simulink model "vehicle_model"  (R2021b)
settings: Solver=ode23tb  StartTime=0  StopTime=181.45  FixedStep=1e-5  RelTol=2e-1
InitFcn:
  | param_v1_script;
  | Ts=0.01;
  | scenario_generator;
  | Regen_on=0;
  | v_nom=10;
  | load('eq_udds.mat')
  | %load('eq_nedc.mat')
values from neighbouring files (symbols this model uses):
  b = 1.504    [dynamics_wheel.m]    (also in param_v1_script.m = Simulink.Parameter)
  BattChargeMax = 4.8    [param_v1_script.m]
  Battery = struct    [param_v1_script.m]
  BattSocInit = 0.75    [param_v1_script.m]
  BattTempInit = 25    [param_v1_script.m]
  BrkPrsMax = 5.0E+6    (= 5000000)    [param_v1_script.m]
  car = vehicle(scenario,'ClassID',1,'Position',[x_ego y_ego 0], 'Yaw' ,0,     'Length',3,'Width',2,'Height',1.6)    [scenario_generator.m]
  curvature = (DX.*D2Y - DY.*D2X) ./(DX.^2+DY.^2).^(3/2)    [ref_generator.m]
  direction = ones(length(gradbp),1)    [ref_generator.m]
  disk_abore = 0.05    [param_v1_script.m]
  Eb_init = 54.28*1000*3600    (= 195408000)    [param_v1_script.m]
  efficiency_table = [86.7 86.7 86.7 86.7 86.7 86.7 86.7 86.7 86.7 86.7 86.7 86.7 86.7 86.7     86.7 ... (first row only)    [param_v1_script.m]
  eta_i = 1    [param_v1_script.m]
  gradbp = distbp    [ref_generator.m]
  Jmotor = Simulink.Parameter    [param_v1_script.m]
  k = Simulink.Parameter    [param_v1_script.m]
  L = 30000    [scenario_generator.m]
  losses_table = [0 0 0 0 0 0 0 0 0 0 0 0 0 0 0 ... (first row only)    [param_v1_script.m]
  m = 3152    [param_v1_script.m]
  MaxChrgCurrLim = Simulink.Parameter    [param_v1_script.m]
  MaxDchrgCurrLim = Simulink.Parameter    [param_v1_script.m]
  MinCellVoltDchrgCurrentLim_BP = [2.5; 2.75; 3]    [param_v1_script.m]
  MinCellVoltDchrgCurrentLim_Table = [0 0.5 1]    [param_v1_script.m]
  MotSpd = [0 1600 3200 4477.56 4800 6400 8000 9600 11200 12800 14400 16000            ]    [param_v1_script.m]
  MotTrq = [450 450 450 450 419.771162404874 314.828371803655 251.862697442924            209.885581202437 179.901926744946 157.414185901828 139.923720801625            125.931348721462]    [param_v1_script.m]
  mu_kinetic = 0.2    [param_v1_script.m]
  Nd = 12    [param_v1_script.m]
  Ndiff = Simulink.Parameter    [param_v1_script.m]
  Np_Module = 31    [param_v1_script.m]
  Ns_Module = 24    [param_v1_script.m]
  num_pads = 2    [param_v1_script.m]
  NumModules = 4    [param_v1_script.m]
  psi_o = thetaRefs(1)*(pi/180)    [ref_generator.m]
  RegenBrkCutOff = [0 1]    [param_v1_script.m]
  RegenBrkSpd_bpt = [5 9]    [param_v1_script.m]
  Rm = 0.177    [param_v1_script.m]
  rw = 0.419    [param_v1_script.m]
  scenario = drivingScenario('SampleTime',0.1','StopTime',60)    [scenario_generator.m]
  SOCInit = 0.75    [param_v1_script.m]
  SOE_init = SOCInit    (= 0.75)    [param_v1_script.m]
  T_eff_bp = [0 32.142857142857146 64.285714285714292 96.428571428571431              128.57142857142858 160.71428571428572 192.85714285714286 225              257.14285714285717 289.28571428571428 321.42857142857144 353.57142857142856              385.71428571428572 417.85714285714283 450]    [param_v1_script.m]
  thetaRefs = smooth(gradbp,thetaRef)    [ref_generator.m]
  threshld = 50    [scenario_generator.m]
  VEH = struct    [dynamics_wheel.m]
  w_eff_bp = [0 1600 3200 4477.56 4800 6400 8000 9600 11200 12800 14400 16000              ]    [param_v1_script.m]
  xRef2s = smooth(gradbp,xRef2)    [ref_generator.m]
  yRef2s = smooth(gradbp,yRef2)    [ref_generator.m]
undefined symbols (not defined in the file or in its folder): DiscIntNeverNeededParam, InertFrm
libraries: simulink x11, autolibsharedcoupling x10, autolibshared x5, autolibutils x4, autolibshareddiff x3, sharedtransform x3, vehdynlibdriver x3, simulink_extras x3, sharedTrackingLibrary x2, vehdynlibtirecommon x2, vehdynlibtire x2, vehdynlibdrivercommon x2
(part 2 of 6)

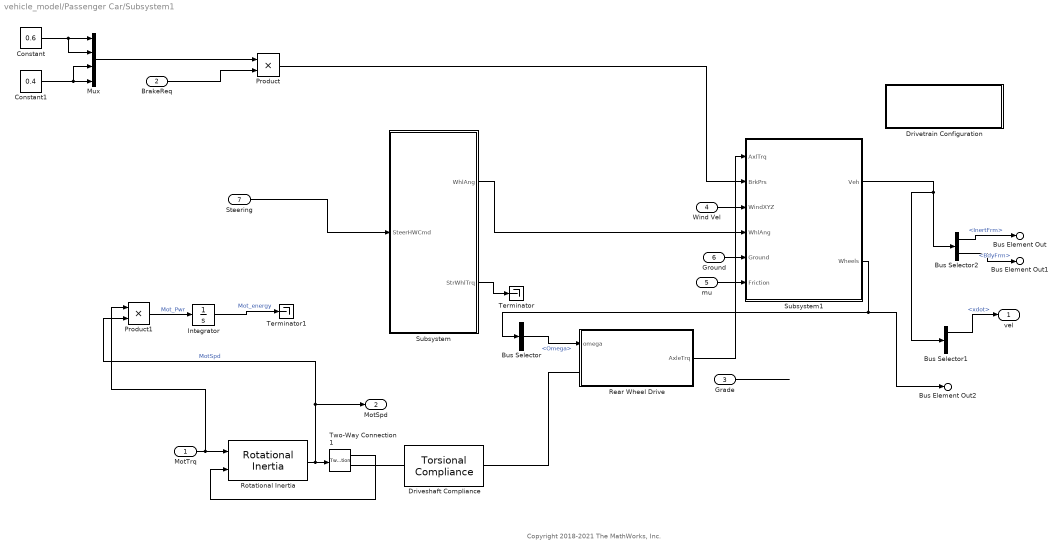
== system vehicle_model/Passenger Car/Subsystem1 ==
  note: Copyright 2018-2021 The MathWorks, Inc.
  MotTrq : Inport
  BrakeReq : Inport  Port=2
  Grade : Inport  Port=3
  Wind Vel : Inport  Port=4
  mu : Inport  Port=5
  Ground : Inport  Port=6
  Steering : Inport  Port=7
  Bus Selector : BusSelector  OutputSignals=TireFrame.Omega
  Bus Selector1 : BusSelector  OutputSignals=BdyFrm.Cg.Vel.xdot,BdyFrm.Cg.Vel.ydot
  Bus Selector2 : BusSelector  OutputSignals=InertFrm,BdyFrm
  Constant : Constant  Value=0.6
  Constant1 : Constant  Value=0.4
  Driveshaft Compliance : autolibsharedcoupling/Torsional Compliance  port_config=Two-way connection  extInfo=off  k=k  b=b  theta_o=theta_o  domega_o=domega_o  omega_c=omega_c  blkID=0  aMode=1
      settings: SourceProductBaseCode=PW,DR,MT,UV,VE
  Drivetrain Configuration : Subsystem  mask(Drivetrain Configuration){drivetrainMode=Rear Wheel Drive}
      mask prompts: drivetrainMode "Drivetrain Mode"
      mask help: Use this block to configure the dirvetrain mode.
      settings: AttributesFormatString=Active Mode: %<drivetrainMode>
      mask TypeOptions drivetrainMode: Front Wheel Drive | Rear Wheel Drive | All Wheel Drive
      mask Callback drivetrainMode:
      | switch get_param(gcb,'drivetrainMode')
      |     case 'Front Wheel Drive'
      |         set_param([bdroot '/Differential and Compliance'],'OverrideUsingVariant','0')
      |     case 'Rear Wheel Drive'
      |         set_param([bdroot '/Differential and Compliance'],'OverrideUsingVariant','1')
      |     case 'All Wheel Drive'
      |         set_param([bdroot '/Differential and Compliance'],'OverrideUsingVariant','2')
      |     otherwise
      |         set_param([bdroot '/Differential and Compliance'],'OverrideUsingVariant','0')
      | end
      mask Display: disp('Double click to configure drivetrain')
  Integrator : Integrator
  Mux : Mux
  Product : Product
  Product1 : Product
  Rear Wheel Drive : Subsystem  VariantControl=0
  Rotational Inertia : autolibsharedcoupling/Rotational Inertia  port_config=Simulink  extInfo=off  externJ=off  J=Jmotor  b=.001  omega_o=omega_o  blkID=0  aMode=1
      settings: SourceProductBaseCode=PW,DR,MT,UV,VE
  Subsystem : Subsystem
  Subsystem1 : Subsystem
  Terminator : Terminator
  Terminator1 : Terminator
  Two-Way Connection1 : TwoWayConnection
  vel : Outport  VectorParamsAs1DForOutWhenUnconnected=off
  MotSpd : Outport  Port=2  VectorParamsAs1DForOutWhenUnconnected=off  BusOutputAsStruct=on
  Bus Element Out : Outport  Port=3  PortName=Veh  Element=InertFrm
  Bus Element Out1 : Outport  Port=3  PortName=Veh  Element=BdyFrm
  Bus Element Out2 : Outport  Port=4  PortName=Wheels  Element=signal1
  wires:
  Subsystem/2(StrWhlTrq) -> Terminator/1
  Bus Selector/1 -> Rear Wheel Drive/1(omega)  "<Omega>"
  Rear Wheel Drive/1(AxleTrq) -> Subsystem1/1(AxlTrq)
  Subsystem1/1(Veh) -> Bus Selector2/1, Bus Selector1/1
  BrakeReq/1 -> Product/2
  Bus Selector2/2 -> Bus Element Out1/1  "<BdyFrm>"
  Steering/1 -> Subsystem/1(SteerHWCmd)
  Product1/1 -> Integrator/1  "Mot_Pwr"
  Product/1 -> Subsystem1/2(BrkPrs)
  MotTrq/1 -> Product1/1, Rotational Inertia/1
  Bus Selector2/1 -> Bus Element Out/1  "<InertFrm>"
  Rotational Inertia/1 -> MotSpd/1, Product1/2, Two-Way Connection1/1  "MotSpd"
  mu/1 -> Subsystem1/6(Friction)
  Bus Selector1/1 -> vel/1  "<xdot>"
  Two-Way Connection1/1 -> Rotational Inertia/2
  Wind Vel/1 -> Subsystem1/3(WindXYZ)
  Ground/1 -> Subsystem1/5(Ground)
  Subsystem1/2(Wheels) -> Bus Element Out2/1, Bus Selector/1
  Mux/1 -> Product/1
  Constant1/1 -> Mux/3, Mux/4
  Constant/1 -> Mux/2, Mux/1
  Grade/1 -> ?
  Subsystem/1(WhlAng) -> Subsystem1/4(WhlAng)
  Integrator/1 -> Terminator1/1  "Mot_energy"
  connections:
  Rear Wheel Drive/LConn1 -- Driveshaft Compliance/RConn1
  Two-Way Connection1/RConn1 -- Driveshaft Compliance/LConn1

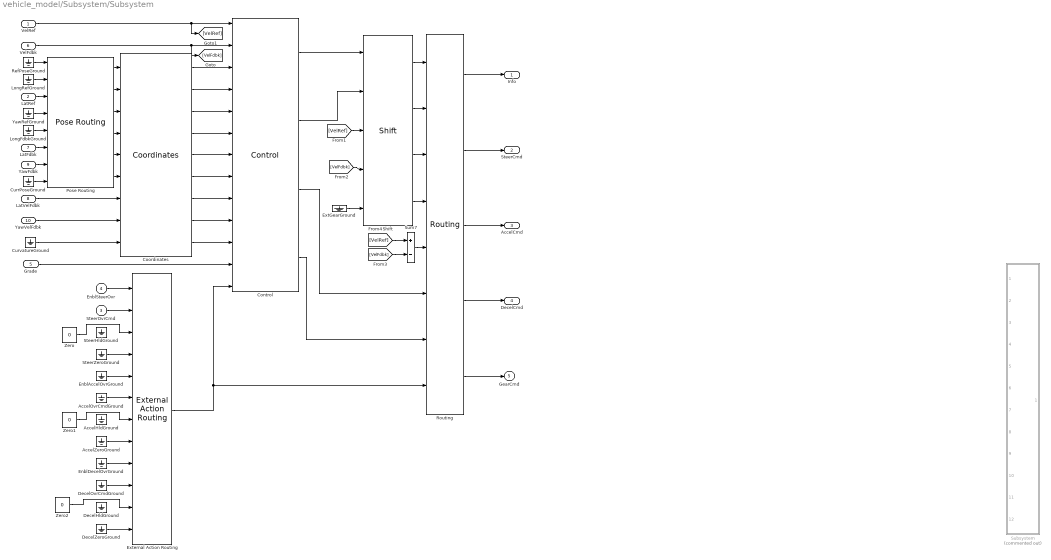
== system vehicle_model/Subsystem/Subsystem ==
  VelRef : Inport  Unit=m/s
  LatRef : Inport  Port=2
  SteerOvrCmd : Inport  Port=3
  EnblSteerOvr : Inport  Port=4
  Grade : Inport  Port=5  Unit=deg
  VelFdbk : Inport  Port=6  Unit=m/s
  LatFdbk : Inport  Port=7
  LatVelFdbk : Inport  Port=8
  YawFdbk : Inport  Port=9
  YawVelFdbk : Inport  Port=10
  AccelHldGround : Ground
  AccelOvrCmdGround : Ground
  AccelZeroGround : Ground
  Control : vehdynlibdriver/Predictive Driver/Control  SystemSampleTime=-1  VariantControl=Variant1  LabelModeActiveChoice=1  VariantActivationTime=update diagram  Latency=0  AutoFrameSizeCalculation=off
      settings: SourceProductBaseCode=VE
  Coordinates : vehdynlibdrivercommon/Coordinates  VariantControl=Choice  LabelModeActiveChoice=0  yawRateUnit=rad/s  curvUnit=rad/m
      settings: SourceProductBaseCode=VE
  CurrPoseGround : Ground
  CurvatureGround : Ground
  DecelHldGround : Ground
  DecelOvrCmdGround : Ground
  DecelZeroGround : Ground
  EnblAccelOvrGround : Ground
  EnblDecelOvrGround : Ground
  ExtGearGround : Ground
  External Action Routing : vehdynlibdriver/Predictive Driver/External Action Routing  SystemSampleTime=-1  VariantActivationTime=update diagram  Latency=0  AutoFrameSizeCalculation=off
      settings: SourceProductBaseCode=VE
  LongFdbkGround : Ground
  LongRefGround : Ground
  Pose Routing : vehdynlibdrivercommon/Pose Routing  VariantControl=Choice  LabelModeActiveChoice=0  Unit=rad
      settings: SourceProductBaseCode=VE
  RefPoseGround : Ground
  Routing : vehdynlibdriver/Predictive Driver/Routing  SystemSampleTime=-1  VariantActivationTime=update diagram  Latency=0  AutoFrameSizeCalculation=off
      settings: SourceProductBaseCode=VE
  Shift : autolibsharedcommon/Longitudinal Driver/Shift  SystemSampleTime=-1  LabelModeActiveChoice=0  VariantActivationTime=update diagram  Latency=0  AutoFrameSizeCalculation=off
      settings: SourceProductBaseCode=PW,DR,MT,UV,VE
  SteerHldGround : Ground
  SteerZeroGround : Ground
  Subsystem : Subsystem  Commented=on
  Sum7 : Sum  Inputs=+-  InputSameDT=on  SaturateOnIntegerOverflow=on  OutDataTypeStr=Inherit: Same as first input
  YawRefGround : Ground
  Zero : Constant  Value=0  OutDataTypeStr=Inherit: Inherit via back propagation
  Zero1 : Constant  Value=0  OutDataTypeStr=Inherit: Inherit via back propagation
  Zero2 : Constant  Value=0  OutDataTypeStr=Inherit: Inherit via back propagation
  Info : Outport  VectorParamsAs1DForOutWhenUnconnected=off
  SteerCmd : Outport  Port=2  VectorParamsAs1DForOutWhenUnconnected=off
  AccelCmd : Outport  Port=3  VectorParamsAs1DForOutWhenUnconnected=off
  DecelCmd : Outport  Port=4  VectorParamsAs1DForOutWhenUnconnected=off
  GearCmd : Outport  Port=5
  wires:
  Shift/3 -> Routing/3
  Shift/2 -> Routing/2
  CurvatureGround/1 -> Coordinates/9
  RefPoseGround/1 -> Pose Routing/1
  Shift/4 -> Routing/4
  Pose Routing/2 -> Coordinates/2
  [VelRef] -> Shift/3
  VelRef/1 -> Control/1, [VelRef]
  Routing/3 -> AccelCmd/1
  Pose Routing/3 -> Coordinates/3
  Control/1 -> Shift/1
  Routing/2 -> SteerCmd/1
  Grade/1 -> Control/12
  AccelOvrCmdGround/1 -> External Action Routing/6
  Control/2 -> Shift/2
  LatRef/1 -> Pose Routing/3
  Sum7/1 -> Routing/5
  [VelFdbk] -> Sum7/2
  [VelRef] -> Sum7/1
  ExtGearGround/1 -> Shift/5
  SteerZeroGround/1 -> External Action Routing/4
  EnblAccelOvrGround/1 -> External Action Routing/5
  Zero/1 -> External Action Routing/3
  Control/3 -> Routing/6
  AccelZeroGround/1 -> External Action Routing/8
  EnblDecelOvrGround/1 -> External Action Routing/9
  Coordinates/3 -> Control/5
  Pose Routing/4 -> Coordinates/4
  Coordinates/8 -> Control/10
  Pose Routing/1 -> Coordinates/1
  Control/4 -> Routing/7
  CurrPoseGround/1 -> Pose Routing/8
  LatFdbk/1 -> Pose Routing/6
  Coordinates/1 -> Control/3
  Routing/4 -> DecelCmd/1
  Coordinates/9 -> Control/11
  DecelZeroGround/1 -> External Action Routing/12
  YawFdbk/1 -> Pose Routing/7
  Pose Routing/5 -> Coordinates/5
  LongFdbkGround/1 -> Pose Routing/5
  Pose Routing/6 -> Coordinates/6
  Zero2/1 -> External Action Routing/11
  YawVelFdbk/1 -> Coordinates/8
  Coordinates/4 -> Control/6
  Coordinates/7 -> Control/9
  Coordinates/5 -> Control/7
  YawRefGround/1 -> Pose Routing/4
  External Action Routing/1 -> Routing/8, Control/13
  SteerOvrCmd/1 -> External Action Routing/2
  Shift/1 -> Routing/1
  Coordinates/6 -> Control/8
  Zero1/1 -> External Action Routing/7
  DecelOvrCmdGround/1 -> External Action Routing/10
  LatVelFdbk/1 -> Coordinates/7
  Routing/5 -> GearCmd/1
  [VelFdbk] -> Shift/4
  Routing/1 -> Info/1
  EnblSteerOvr/1 -> External Action Routing/1
  Coordinates/2 -> Control/4
  LongRefGround/1 -> Pose Routing/2
  VelFdbk/1 -> Control/2, [VelFdbk]

== system vehicle_model/Visualization/Performance Calculations ==
  BattPwr : Inport
  VehSpd : Inport  Port=2
  Divide : Product  Inputs=*/
  Divide1 : Product  Inputs=*/
  Divide2 : Product  Inputs=*/
  Integrator : Integrator
  Integrator1 : Integrator
  L/100 Km Calc : Product  Inputs=/*
  Product : Product
  Saturation : Saturate  UpperLimit=Inf  LowerLimit=0.001  ZeroCross=off
  Saturation1 : Saturate  UpperLimit=Inf  LowerLimit=1e-3  ZeroCross=off
  Sqrt : Sqrt  SaturateOnIntegerOverflow=on
  US EPA kwh/USgal equivalent : Constant  Value=33.7
  US MPG Calc : Product  Inputs=*/
  m to 100Km : Gain  Gain=1/1000/100
  m to mile : Gain  Gain=0.000621371
  m^3 per gal : Gain  Gain=0.00378541
  m^3 to L : Gain  Gain=1000
  m^3 to US Gal : Gain  Gain=264.172
  s per h : Constant  Value=3600
  w per kw : Constant  Value=1000
  US MPG : Outport  VectorParamsAs1DForOutWhenUnconnected=off
  L/100Km : Outport  Port=2  VectorParamsAs1DForOutWhenUnconnected=off
  wires:
  m^3 to US Gal/1 -> Saturation1/1
  m^3 to L/1 -> L/100 Km Calc/2
  Integrator/1 -> m to mile/1, m to 100Km/1
  m to mile/1 -> US MPG Calc/1
  Integrator1/1 -> m^3 to US Gal/1, m^3 to L/1
  Saturation/1 -> L/100 Km Calc/1
  m to 100Km/1 -> Saturation/1
  L/100 Km Calc/1 -> L/100Km/1  "L/100Km"
  Saturation1/1 -> US MPG Calc/2
  US MPG Calc/1 -> US MPG/1  "US MPG"
  w per kw/1 -> Divide/2
  Divide/1 -> Divide2/1
  Divide2/1 -> Divide1/1
  s per h/1 -> Divide1/2
  Divide1/1 -> m^3 per gal/1
  m^3 per gal/1 -> Integrator1/1
  US EPA kwh/USgal equivalent/1 -> Divide2/2
  BattPwr/1 -> Divide/1
  Sqrt/1 -> Integrator/1
  Product/1 -> Sqrt/1
  VehSpd/1 -> Product/2, Product/1

== system vehicle_model/Visualization/Performance Calculations1 ==
  BattPwr : Inport
  VehSpd : Inport  Port=2
  Divide : Product  Inputs=*/
  Divide1 : Product  Inputs=*/
  Divide2 : Product  Inputs=*/
  Integrator : Integrator
  Integrator1 : Integrator
  L/100 Km Calc : Product  Inputs=/*
  Product : Product
  Saturation : Saturate  UpperLimit=Inf  LowerLimit=0.001  ZeroCross=off
  Saturation1 : Saturate  UpperLimit=Inf  LowerLimit=1e-3  ZeroCross=off
  Sqrt : Sqrt  SaturateOnIntegerOverflow=on
  US EPA kwh/USgal equivalent : Constant  Value=33.7
  US MPG Calc : Product  Inputs=*/
  m to 100Km : Gain  Gain=1/1000/100
  m to mile : Gain  Gain=0.000621371
  m^3 per gal : Gain  Gain=0.00378541
  m^3 to L : Gain  Gain=1000
  m^3 to US Gal : Gain  Gain=264.172
  s per h : Constant  Value=3600
  w per kw : Constant  Value=1000
  US MPG : Outport  VectorParamsAs1DForOutWhenUnconnected=off
  L/100Km : Outport  Port=2  VectorParamsAs1DForOutWhenUnconnected=off
  wires:
  m^3 to US Gal/1 -> Saturation1/1
  m^3 to L/1 -> L/100 Km Calc/2
  Integrator/1 -> m to mile/1, m to 100Km/1
  m to mile/1 -> US MPG Calc/1
  Integrator1/1 -> m^3 to US Gal/1, m^3 to L/1
  Saturation/1 -> L/100 Km Calc/1
  m to 100Km/1 -> Saturation/1
  L/100 Km Calc/1 -> L/100Km/1  "L/100Km"
  Saturation1/1 -> US MPG Calc/2
  US MPG Calc/1 -> US MPG/1  "US MPG"
  w per kw/1 -> Divide/2
  Divide/1 -> Divide2/1
  Divide2/1 -> Divide1/1
  s per h/1 -> Divide1/2
  Divide1/1 -> m^3 per gal/1
  m^3 per gal/1 -> Integrator1/1
  US EPA kwh/USgal equivalent/1 -> Divide2/2
  BattPwr/1 -> Divide/1
  Sqrt/1 -> Integrator/1
  Product/1 -> Sqrt/1
  VehSpd/1 -> Product/2, Product/1

== system vehicle_model/Visualization1/3D Engine ==
  note: 1) Add Subsystem or Model blocks as valid variant choices.
      | 2) You cannot connect blocks at this level. At simulation, connectivity is automatically
      | determined, based on the active variant and port name matching.
  VehFdbk : Inport
  3D Engine : Subsystem  VariantControl=engine3D==1
  3D Engine Disabled : Subsystem  VariantControl=engine3D==2

== system vehicle_model/Visualization1/ISO 15037-1:2006 ==
  VehFdbk : Inport
  Disabled : Subsystem  VariantControl=0
  Enabled : Subsystem  VariantControl=1

== system vehicle_model/lateral controller/Reference Data ==
  note: Select method to calculate theta
  long_ref : Inport
  VelFdbk : Inport  Port=2
  Curvature : Lookup_n-D  NumberOfTableDimensions=1  BreakpointsForDimension1=gradbp  Table=curvature  InternalRulePriority=Speed  RndMeth=Simplest  InputSameDT=on
  Delay : Delay  DelayLength=1
  Direction : Lookup_n-D  NumberOfTableDimensions=1  BreakpointsForDimension1=gradbp  Table=direction  InternalRulePriority=Speed  RndMeth=Simplest  InputSameDT=on
  Integrator : Integrator
  Mux : Mux  Inputs=3
  Switch : Switch  Criteria=u2 > Threshold
  Theta : Subsystem  Variant=on  VariantControlMode=label  LabelModeActiveChoice=thetaSimulinkBlock
  X Ref : Lookup_n-D  NumberOfTableDimensions=1  BreakpointsForDimension1=gradbp  Table=xRef2s  InternalRulePriority=Speed  RndMeth=Simplest  InputSameDT=on
  Y Ref : Lookup_n-D  NumberOfTableDimensions=1  BreakpointsForDimension1=gradbp  Table=yRef2s  InternalRulePriority=Speed  RndMeth=Simplest  InputSameDT=on
  RefPose : Outport
  DirectionO : Outport  Port=2
  CurvatureO : Outport  Port=3
  tag scope: xRef=global, yRef=global
  wires:
  Direction/1 -> DirectionO/1
  Curvature/1 -> CurvatureO/1
  Switch/1 -> Delay/1, Mux/2, [yRef], Theta/1(y)  "y_ref"
  Mux/1 -> RefPose/1
  X Ref/1 -> Theta/2(x), Mux/1, [xRef]
  Integrator/1 -> Curvature/1, Direction/1, X Ref/1, Y Ref/1, Theta/3(dis)
  VelFdbk/1 -> Integrator/1
  Theta/1(theta) -> Mux/3
  Y Ref/1 -> Switch/1  "y_ref"
  Delay/1 -> Switch/3
  long_ref/1 -> Switch/2

== system vehicle_model/lateral controller/Subsystem ==
  VehFdbk : Inport
  Bus Selector : BusSelector  OutputSignals=Body.InertFrm.Cg.Disp.X,Body.InertFrm.Cg.Disp.Y,Body.InertFrm.Cg.Ang.psi
  Gain1 : Gain  Gain=180/pi
  Mux : Mux  Inputs=3
  Transpose : Math  Operator=transpose  SignedPower=on  SaturateOnIntegerOverflow=on
  pose : Outport
  wires:
  Mux/1 -> Transpose/1
  VehFdbk/1 -> Bus Selector/1
  Bus Selector/1 -> Mux/1  "<X>"
  Gain1/1 -> Mux/3
  Bus Selector/2 -> Mux/2  "<Y>"
  Transpose/1 -> pose/1
  Bus Selector/3 -> Gain1/1  "<psi>"

== system vehicle_model/Controllers/Powertrain Control Module (PCM)/Subsystem ==
  Sensors : Inport  OutDataTypeStr=Bus: Sensors  BusOutputAsStruct=on
  Subsystem : Subsystem
  Subsystem1 : Subsystem
  Subsystem4 : Subsystem
  Unit Delay : UnitDelay  InitialCondition=struct('Cell_Voltages',3.6*ones(1, Ns_Module*NumModules),'Pack_Voltage',3.6*Ns_Module*NumModules,'Pack_Current',0,'Cell_Temperatures',BattTempInit*ones(1,Ns_Module*NumModules),'Vout_Chgr',0,'Vout_Invtr',0)  SampleTime=-1  HasFrameUpgradeWarning=on
  BMS_Info : Outport  OutDataTypeStr=Bus: SOC_Est  VectorParamsAs1DForOutWhenUnconnected=off
  BMS_Cmd : Outport  Port=2  OutDataTypeStr=Bus: CurrentLimits  VectorParamsAs1DForOutWhenUnconnected=off  BusOutputAsStruct=on
  wires:
  Subsystem4/1(BMS_Info) -> BMS_Info/1
  Unit Delay/1 -> Subsystem/1(Sensors), [Sensors]
  [Sensors] -> Subsystem1/1(Sensors)
  Subsystem/1(CurrentLimits) -> Subsystem4/2(CurrentLimits)
  Sensors/1 -> Unit Delay/1
  Subsystem4/2(BMS_Commands) -> BMS_Cmd/1
  Subsystem1/1(SOC) -> Subsystem4/1(SOC)

== system vehicle_model/Controllers/Powertrain Control Module (PCM)/Subsystem1 ==
  note: Copyright 2015-2018 The MathWorks, Inc.
  AccCmd : Inport
  DecCmd : Inport  Port=2  OutDataTypeStr=double
  VehSpdFdbk : Inport  Port=3
  Batt_Info : Inport  Port=4  OutDataTypeStr=Bus: SOC_Est
  BMS_Cmd : Inport  Port=5  OutDataTypeStr=Bus: CurrentLimits
  MotSpd : Inport  Port=6
  BMS_Sensors : Inport  Port=7  OutDataTypeStr=Bus: Sensors
  Accel Pedal to Traction Wheel Torque Request : Subsystem
  Brake Pedal to Total Braking Pressure Request : Subsystem
  Constant : Constant  Value=0
  Motor Torque Arbitration and Power Management : Subsystem
  Power Limit Calculations : Subsystem
  Rate Transition : RateTransition
  Rate Transition1 : RateTransition
  Series Regen Braking : Subsystem  InitFcn=%[~]=autosharedicon('autolibutils',gcb,0);  VariantControl=Variant
  Subsystem2 : Subsystem
  MotTrqCmd : Outport  VectorParamsAs1DForOutWhenUnconnected=off
  BrakeCmd : Outport  Port=2  VectorParamsAs1DForOutWhenUnconnected=off
  wires:
  [MotSpd] -> Motor Torque Arbitration and Power Management/5(MotSpd)
  BMS_Cmd/1 -> Rate Transition/1
  Power Limit Calculations/2(BattPwrChrgLmt) -> Motor Torque Arbitration and Power Management/4("BattPwrChrgLmt ")  "BattPwrChrgLmt"
  [MotTrqCmd] -> Series Regen Braking/4(MotTrqCmdFinal)
  Power Limit Calculations/1(BattPwrDischrgLmt) -> Motor Torque Arbitration and Power Management/3(BattPwrDisChrgLmt)  "BattPwrDischrgLmt"
  Series Regen Braking/1(" MotTrqCmdRegen") -> Motor Torque Arbitration and Power Management/7(MotTrqCmdRegen)  "MotTrqCmdRegen"
  Accel Pedal to Traction Wheel Torque Request/1(TrqCmd) -> Motor Torque Arbitration and Power Management/1(MotTrqCmdTrac)
  Motor Torque Arbitration and Power Management/1(MotTrqCmdFinal) -> [MotTrqCmd], MotTrqCmd/1  "MotTrqCmd"
  Batt_Info/1 -> Rate Transition1/1  "SOC"
  DecCmd/1 -> Brake Pedal to Total Braking Pressure Request/1(DecelPdl)  "DecelPdl"
  [MotSpd] -> Accel Pedal to Traction Wheel Torque Request/2(MotSpd)
  BMS_Sensors/1 -> Power Limit Calculations/2(BMS_Sensors)
  Subsystem2/1(BattSOC) -> Motor Torque Arbitration and Power Management/6(SOC)  "SOC"
  Constant/1 -> Brake Pedal to Total Braking Pressure Request/2(Park)
  MotSpd/1 -> Series Regen Braking/2(MotSpd), [MotSpd]  "MotSpd"
  AccCmd/1 -> [AccelPdl], Accel Pedal to Traction Wheel Torque Request/1(AccelPdl)
  Brake Pedal to Total Braking Pressure Request/1(BrkPrsReq) -> Series Regen Braking/3("BrkPrsReq ")
  [AccelPdl] -> Motor Torque Arbitration and Power Management/2(AccelPdl)
  Series Regen Braking/2(" BrkCmd") -> BrakeCmd/1  "BrkCmd"
  VehSpdFdbk/1 -> Series Regen Braking/1(VehSpd)  "VehSpd"
  Rate Transition/1 -> Power Limit Calculations/1(BMS_Cmd)
  Rate Transition1/1 -> Subsystem2/1(BMS_info)

== system vehicle_model/Passenger Car/Subsystem/Accessory Load ==
  BattV : Inport
  Accessory Load W : Constant  Value=0
  Divide : Product  Inputs=*/
  div0protect - poly : autolibutils/div0protect - poly  thresh=.01  ZeroCross=off  ZeroCross1=off  aMode=aMode
      settings: SourceProductBaseCode=PW,DR,MT,UV,VE
  Accessory Current : Outport
  wires:
  BattV/1 -> div0protect - poly/1
  Accessory Load W/1 -> Divide/1
  Divide/1 -> Accessory Current/1
  div0protect - poly/1 -> Divide/2

== system vehicle_model/Passenger Car/Subsystem/BMS Signal Creation ==
  note: Create signal vectors
      | matching number of
      | cells in series for
      | detailed batteries
  note: BMS has opposite
      | sign convention
  BattV : Inport
  BattTmp : Inport  Port=2
  BattCrnt : Inport  Port=3
  Bus Creator : BusCreator  Inputs=6  OutDataTypeStr=Bus: Sensors  NonVirtualBus=on
      settings: InheritFromInputs=off
  Constant : Constant  Value=0
  Convert K to degC : Subsystem
  Data Type Conversion{1..5} (5 alike) : DataTypeConversion  OutDataTypeStr=single
  Gain : Gain  Gain=ones(96,1)./96
  Gain1 : Gain  Gain=ones(96,1)
  Gain2 : Gain  Gain=-1
  BMS_Sensors : Outport
  wires:
  Gain1/1 -> Bus Creator/4  "Cell_Temperatures"
  Data Type Conversion4/1 -> Bus Creator/5  "Vout_Chgr"
  Gain2/1 -> Bus Creator/3  "Pack_Current"
  Data Type Conversion5/1 -> Bus Creator/6  "Vout_Invtr"
  Data Type Conversion2/1 -> Gain2/1
  Gain/1 -> Bus Creator/1  "Cell_Voltages"
  Data Type Conversion3/1 -> Gain1/1
  Data Type Conversion1/1 -> Gain/1, Bus Creator/2  "Pack_Voltage"
  BattTmp/1 -> Convert K to degC/1(In1)
  BattCrnt/1 -> Data Type Conversion2/1
  Constant/1 -> Data Type Conversion4/1
  BattV/1 -> Data Type Conversion1/1, Data Type Conversion5/1
  Bus Creator/1 -> BMS_Sensors/1  "BMS_Sensors"
  Convert K to degC/1(Out1) -> Data Type Conversion3/1

== system vehicle_model/Passenger Car/Subsystem/Subsystem ==
  BattCrnt : Inport
  BattTemp : Inport  Port=2
  Lithium Ion Battery Pack : autolibdatasheetbattery/Datasheet Battery  CapacityCtrl=Parameter  OutputVlt=Unfiltered  BattChargeMax=BattChargeMax  Em=Em  CapLUTBp=CapLUTBp  RInt=RInt  BattTempBp=BattTempBp  CapSOCBp=CapSOCBp  Ns=Ns  Np=Np  BattCapInit=BattChargeMax*BattSocInit  Tc=1/1000  Vinit=3.75*72  RefBlkName='autolibdatasheetbattery/Datasheet Battery'
      settings: SourceProductBaseCode=PW
  Terminator : Terminator
  BattV : Outport  VectorParamsAs1DForOutWhenUnconnected=off
  wires:
  Lithium Ion Battery Pack/1 -> Terminator/1
  BattTemp/1 -> Lithium Ion Battery Pack/2
  Lithium Ion Battery Pack/2 -> BattV/1
  BattCrnt/1 -> Lithium Ion Battery Pack/1

== system vehicle_model/Passenger Car/Subsystem/Subsystem1 ==
  MotTrqCmd : Inport
  MotSpd : Inport  Port=2
  BusVolt : Inport  Port=3
  Bus Selector : BusSelector  OutputSignals=PwrLoss
  Mapped Motor : autolibmappedmotor/Mapped Motor  port_config=Speed  param_by=Maximum torque and power  w_t=[ 0 375 750 800 ]  T_t=[0.09 0.08 0.07 0]  torque_max=torque_max  power_max=power_max  Tc=Tc  param_loss=Tabulated efficiency data  eff=100  w_eff=375  T_eff=0.08  Piron=0  Pbase=0  w_eff_bp=w_eff_bp.*pi/30  T_eff_bp=T_eff_bp  Temp_eff_bp=[233.15 293.15 373.15]  losses_table=losses_table  losses_table_3d=cat(3,losses_table,losses_table,losses_table)  efficiency_table=efficiency_table  efficiency_table_3d=cat(3,efficiency_table,efficiency_table,efficiency_table)  J=5e-6  b=1e-5  omega_o=0  T_t_extended=[0 0.07 0.08 0.09 0.08 0.07 0]  w_t_extended=[-800 -750 -375 0 375 750 800]  KLossIron=0  KLossCopper=0  x_w_eff_vec=[-1675.51608191456 -1507.9644737231 -1340.41286553165 -1172.86125734019 -1005.30964914873 -837.758040957278 -670.206432765823 -502.654824574367 -468.888986733584 -335.103216382911 -167.551608191456 0 167.551608191456 335.103216382911 468.888986733584 502.654824574367 670.206432765823 837.758040957278 1005.30964914873 1172.86125734019 1340.41286553165 1507.9644737231 1675.51608191456]  x_T_eff_vec=[-450 -417.857142857143 -385.714285714286 -353.571428571429 -321.428571428571 -289.285714285714 -257.142857142857 -225 -192.857142857143 -160.714285714286 -128.571428571429 -96.4285714285714 -64.2857142857143 -32.1428571428571 0 32.1428571428571 64.2857142857143 96.4285714285714 128.571428571429 160.714285714286 192.857142857143 225 257.142857142857 289.285714285714 321.428571428571 353.571428571429 385.714285714286 417.857142857143 450]  x_tmp_eff_vec=[233.15 293.15 373.15]  x_losses_mat=[40854.6141415599 37936.4274171628 35018.2406927657 32100.0539683685 29181.8672439714 26263.6805195742 23345.4937951771 20427.30707078 17509.1203463828 14590.9336219857 11672.7468975886 10605.888242298 9621.31083452336 8261.6277395441 0 7162.83125018473 8832.36334609244 9952.56552657246 11072.7677070525 13840.9596338156 16609.1515605787 19377.3434873418 22145.535414105 24913.7273408681 27681.9192676312 30450.1111943943 33218.3031211574 35986.4950479206 38754.6869746837;29159.0126646081 27076.2260457076 24993.439426807 22910.6528079064 20827.8661890058 18745.0795701052 16662.2929512047 14579.5063323041 12496.7197134035 10413.9330945029 8331.14647560233 6248.35985670175 5252.73610391485 7435.46496558969 0 6446.54812516626 4982.74546817362 5990.92743060563 7987.90324080751 9984.87905100939 11981.8548612113 13978.8306714131 15975.806481615 17972.7822918169 19969.7581020188 21966.7339122207 23963.7097224225 25960.6855326244 27957.6613428263;19296.9654016165 17918.6107300724 16540.2560585284 15161.9013869844 13783.5467154403 12405.1920438963 11026.8373723523 9648.48270080824 8270.1280292642 6891.77335772017 5513.41868617614 5554.09765040155 4669.09875903542 6609.30219163528 0 5730.26500014778 4429.10708282099 5325.26882720501 5342.50270690469 6678.12838363086 8013.75406035703 9349.3797370832 10685.0054138094 12020.6310905355 13356.2567672617 14691.8824439879 16027.5081207141 17363.1337974402 18698.7594741664;16884.8447264144 15678.7843888134 14472.7240512124 13266.6637136113 12060.6033760103 10854.5430384093 9648.48270080824 8442.4223632072 7236.36202560618 6030.30168800515 4824.24135040412 4859.83544410136 4085.46141415599 5783.13941768087 0 5013.98187512931 3875.46869746837 4659.61022380438 4674.6898685416 5843.362335677 7012.0348028124 8180.7072699478 9349.3797370832 10518.0522042186 11686.724671354 12855.3971384894 14024.0696056248 15192.7420727602 16361.4145398956;14472.7240512124 13438.9580475543 12405.1920438963 11371.4260402383 10337.6600365803 9303.89403292223 8270.1280292642 7236.36202560618 6202.59602194815 5168.83001829013 5554.09765040155 4165.57323780116 3501.82406927657 4956.97664372646 0 4297.69875011084 3321.83031211575 3993.95162040376 5325.26882720501 5008.59628772314 6010.31554526777 7012.0348028124 8013.75406035703 9015.47331790166 10017.1925754463 11018.9118329909 12020.6310905355 13022.3503480802 14024.0696056248;12060.6033760103 11199.1317062953 10337.6600365803 9476.18836686523 8614.71669715021 7753.24502743519 6891.77335772017 6030.30168800515 5168.83001829013 4307.35834857511 4628.41470866796 3471.31103150097 2918.18672439714 4130.81386977205 0 3581.41562509236 2768.19192676312 3328.29301700313 4437.72402267084 4173.83023976929 5008.59628772314 5843.362335677 6678.12838363086 7512.89443158471 8347.66047953857 9182.42652749243 10017.1925754463 10851.9586234001 11686.724671354;12959.5611842703 12033.8782425367 11108.1953008031 10182.5123590695 9256.82941733592 8331.14647560233 7405.46353386874 6479.78059213514 5554.09765040155 4628.41470866796 3702.73176693437 2777.04882520078 2334.54937951771 3304.65109581764 0 2865.13250007389 2214.5535414105 2662.6344136025 3550.17921813667 4437.72402267084 5325.26882720501 6212.81363173918 7100.35843627335 7987.90324080751 8875.44804534168 9762.99284987585 10650.53765441 11538.0824589442 12425.6272634784;20204.7527524991 18761.5561273206 17318.359502142 15875.1628769635 10605.888242298 9545.29941806823 8484.71059383843 6128.19212123399 5252.73610391485 4377.28008659571 3501.82406927657 3181.76647268941 2121.17764845961 2478.48832186323 0 2148.84937505542 1990.51310531449 2985.76965797174 3321.83031211575 4152.28789014468 4982.74546817362 5813.20304620255 7962.05242125797 8957.30897391522 9952.56552657246 14573.3995210525 15898.2540229664 17223.1085248803 18547.9630267941;18847.4984863499 17501.2485944678 16154.9987025857 14808.7488107035 9893.43769962166 8904.0939296595 7914.75015969733 6925.40638973516 5936.062619773 4946.71884981083 3957.37507984867 2968.0313098865 ...(+6504 chars)]  x_losses_mat_3d=cat(3,[93 93 93 93 93 93 93 93 93 93 93 92 90 85 85 85 90 92 93 93 93 93 93 93 93 93 93 93 93;94 94 94 94 94 94 94 94 94 94 94 94 93 85 85 85 93 94 94 94 94 94 94 94 94 94 94 94 94;95 95 95 95 95 95 95 95 95 95 95 94 93 85 85 85 93 94 95 95 95 95 95 95 95 95 95 95 95;95 95 95 95 95 95 95 95 95 95 95 94 93 85 85 85 93 94 95 95 95 95 95 95 95 95 95 95 95;95 95 95 95 95 95 95 95 95 95 94 94 93 85 85 85 93 94 94 95 95 95 95 95 95 95 95 95 95;95 95 95 95 95 95 95 95 95 95 94 94 93 85 85 85 93 94 94 95 95 95 95 95 95 95 95 95 95;94 94 94 94 94 94 94 94 94 94 94 94 93 85 85 85 93 94 94 94 94 94 94 94 94 94 94 94 94;90 90 90 90 92 92 92 93 93 93 93 92 92 85 85 85 92 92 93 93 93 93 92 92 92 90 90 90 90;90 90 90 90 92 92 92 92 92 92 92 92 92 85 85 85 92 92 92 92 92 92 92 92 92 90 90 90 90;88 88 88 88 88 90 90 90 90 90 90 90 90 85 85 85 90 90 90 90 90 90 90 90 88 88 88 88 88;85 85 85 85 85 85 85 85 85 85 85 85 85 85 85 85 85 85 85 85 85 85 85 85 85 85 85 85 85;85 85 85 85 85 85 85 85 85 85 85 85 85 85 85 85 85 85 85 85 85 85 85 85 85 85 85 85 85;85 85 85 85 85 85 85 85 85 85 85 85 85 85 85 85 85 85 85 85 85 85 85 85 85 85 85 85 85;88 88 88 88 88 90 90 90 90 90 90 90 90 85 85 85 90 90 90 90 90 90 90 90 88 88 88 88 88;90 90 90 90 92 92 92 92 92 92 92 92 92 85 85 85 92 92 92 92 92 92 92 92 92 90 90 90 90;90 90 90 90 92 92 92 93 93 93 93 92 92 85 85 85 92 92 93 93 93 93 92 92 92 90 90 90 90;94 94 94 94 94 94 94 94 94 94 94 94 93 85 85 85 93 94 94 94 94 94 94 94 94 94 94 94 94;95 95 95 95 95 95 95 95 95 95 94 94 93 85 85 85 93 94 94 95 95 95 95 95 95 95 95 95 95;95 95 95 95 95 95 95 95 95 95 94 94 93 85 85 85 93 94 94 95 95 95 95 95 95 95 95 95 95;95 95 95 95 95 95 95 95 95 95 95 94 93 85 85 85 93 94 95 95 95 95 95 95 95 95 95 95 95;95 95 95 95 95 95 95 95 95 95 95 94 93 85 85 85 93 94 95 95 95 95 95 95 95 95 95 95 95;94 94 94 94 94 94 94 94 94 94 94 94 93 85 85 85 93 94 94 94 94 94 94 94 94 94 94 94 94;93 93 93 93 93 93 93 93 93 93 93 92 90 85 85 85 90 92 93 93 93 93 93 93 93 93 93 93 93],[93 93 93 93 93 93 93 93 93 93 93 92 90 85 85 85 90 92 93 93 93 93 93 93 93 93 93 93 93;94 94 94 94 94 94 94 94 94 94 94 94 93 85 85 85 93 94 94 94 94 94 94 94 94 94 94 94 94;95 95 95 95 95 95 95 95 95 95 95 94 93 85 85 85 93 94 95 95 95 95 95 95 95 95 95 95 95;95 95 95 95 95 95 95 95 95 95 95 94 93 85 85 85 93 94 95 95 95 95 95 95 95 95 95 95 95;95 95 95 95 95 95 95 95 95 95 94 94 93 85 85 85 93 94 94 95 95 95 95 95 95 95 95 95 95;95 95 95 95 95 95 95 95 95 95 94 94 93 85 85 85 93 94 94 95 95 95 95 95 95 95 95 95 95;94 94 94 94 94 94 94 94 94 94 94 94 93 85 85 85 93 94 94 94 94 94 94 94 94 94 94 94 94;90 90 90 90 92 92 92 93 93 93 93 92 92 85 85 85 92 92 93 93 93 93 92 92 92 90 90 90 90;90 90 90 90 92 92 92 92 92 92 92 92 92 85 85 85 92 92 92 92 92 92 92 92 92 90 90 90 90;88 88 88 88 88 90 90 90 90 90 90 90 90 85 85 85 90 90 90 90 90 90 90 90 88 88 88 88 88;85 85 85 85 85 85 85 85 85 85 85 85 85 85 85 85 85 85 85 85 85 85 85 85 85 85 85 85 85;85 85 85 85 85 85 85 85 85 85 85 85 85 85 85 85 85 85 85 85 85 85 85 85 85 85 85 85 85;85 85 85 85 85 85 85 85 85 85 85 85 85 85 85 85 85 85 85 85 85 85 85 85 85 85 85 85 85;88 88 88 88 88 90 90 90 90 90 90 90 90 85 85 85 90 90 90 90 90 90 90 90 88 88 88 88 88;90 90 90 90 92 92 92 92 92 92 92 92 92 85 85 85 92 92 92 92 92 92 92 92 92 90 90 90 90;90 90 90 90 92 92 92 93 93 93 93 92 92 85 85 85 92 92 93 93 93 93 92 92 92 90 90 90 90;94 94 94 94 94 94 94 94 94 94 94 94 93 85 85 85 93 94 94 94 94 94 94 94 94 94 94 94 94;95 95 95 95 95 95 95 95 95 95 94 94 93 85 85 85 93 94 94 95 95 95 95 95 95 95 95 95 95;95 95 95 95 95 95 95 95 95 95 94 94 93 85 85 85 93 94 94 95 95 95 95 95 95 95 95 95 95;95 95 95 95 95 95 95 95 95 95 95 94 93 85 85 85 93 94 95 95 95 95 95 95 95 95 95 95 95;95 95 95 95 95 95 95 95 95 95 95 94 93 85 85 85 93 94 95 95 95 95 95 95 95 95 95 95 95;94 94 94 94 94 94 94 94 94 94 94 94 93 85 85 85 93 94 94 94 94 94 94 94 94 94 94 94 94;93 93 93 93 93 93 93 93 93 93 93 92 90 85 85 85 90 92 93 93 93 93 93 93 93 93 ...(+2012 chars)])  CalLossMapData={}  CalLossWithTempMapData={}  aMode=aMode  RefBlkName='autolibmappedmotor/Mapped Motor'
      settings: SourceProductBaseCode=PW,DR,MT,UV,VE
  Terminator : Terminator
  MotTrq : Outport  VectorParamsAs1DForOutWhenUnconnected=off
  MotCurnt : Outport  Port=2  VectorParamsAs1DForOutWhenUnconnected=off
  wires:
  Mapped Motor/1 -> Bus Selector/1
  Mapped Motor/2 -> MotCurnt/1
  MotTrqCmd/1 -> Mapped Motor/3
  Mapped Motor/3 -> MotTrq/1
  MotSpd/1 -> Mapped Motor/2
  BusVolt/1 -> Mapped Motor/1
  Bus Selector/1 -> Terminator/1  "<PwrLoss>"

== system vehicle_model/Passenger Car/Subsystem/Subsystem2 ==
  Input : Inport
  Bus Selector : BusSelector  OutputSignals=SOC_CC
  Data Type Conversion : DataTypeConversion
  Rate Transition : RateTransition  Commented=through  InitialCondition=Battery.SOCInit
  convert2percent : Gain  Gain=100
  BattSOC : Outport
  wires:
  convert2percent/1 -> Data Type Conversion/1
  Bus Selector/1 -> convert2percent/1  "<SOC_CC>"
  Data Type Conversion/1 -> Rate Transition/1
  Rate Transition/1 -> BattSOC/1
  Input/1 -> Bus Selector/1

== system vehicle_model/Passenger Car/Subsystem/Temp Selection ==
  AmbTmp : Inport
  Constant : Constant  Value=25
  Convert degC to K : Subsystem
  Manual Switch : ManualSwitch  CurrentSetting=0
  BattTmp : Outport
  wires:
  AmbTmp/1 -> Manual Switch/1
  Manual Switch/1 -> BattTmp/1
  Constant/1 -> Convert degC to K/1(In1)
  Convert degC to K/1(Out1) -> Manual Switch/2

== system vehicle_model/Passenger Car/Subsystem1/Drivetrain Configuration ==
